simulink model "Stiff_RLC_ClosedLoop_Reference"  (R2023a)
settings: Solver=ode4  StartTime=0.0  StopTime=2  FixedStep=0.0005  RelTol=1e-3
settings Model: Creator=Fasih  LastModifiedBy=Fasih

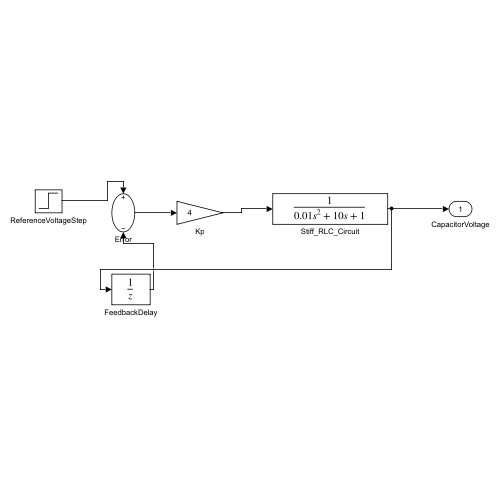
[thumbnail: Simulink's stored preview of the top-level diagram]
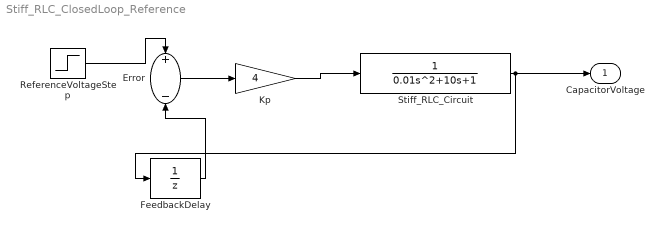
== system Stiff_RLC_ClosedLoop_Reference ==
  Error : Sum  Inputs=+-
  FeedbackDelay : UnitDelay  SampleTime=0.0005  HasFrameUpgradeWarning=on
  Kp : Gain  Gain=4
  ReferenceVoltageStep : Step  Time=0  SampleTime=0
  Stiff_RLC_Circuit : TransferFcn  Numerator=1  Denominator=[0.01 10 1]
  CapacitorVoltage : Outport
  wires:
  ReferenceVoltageStep/1 -> Error/1
  FeedbackDelay/1 -> Error/2
  Error/1 -> Kp/1
  Kp/1 -> Stiff_RLC_Circuit/1
  Stiff_RLC_Circuit/1 -> CapacitorVoltage/1, FeedbackDelay/1
